simulink model "HW_7_2_1B"  (R2019b)
settings: Solver=VariableStepAuto  StartTime=0.0  StopTime=50  RelTol=1e-3  EnableMultiTasking=on
settings Model: Creator=Teng-Hu  LastModifiedBy=liu
settings DataIOCC: ReturnWorkspaceOutputs=off
settings OptimizationCC: LifeSpan=inf
settings DebuggingCC: SFUnexpectedBacktrackingDiag=warning  SFNoUnconditionalDefaultTransitionDiag=warning  SFExecutionAtInitializationDiag=none  ArithmeticOperatorsInVariantConditions=warning
settings SFSimCC: SimUseLocalCustomCode=off  CustomCodeUndefinedFunction=UseInterfaceOnly
settings RTWCC: RTWUseLocalCustomCode=off
settings CodeAppCC: StateflowObjectComments=on
settings GRTTargetCC: TargetLangStandard=C89/C90 (ANSI)
settings ConfigComp: CovMetricSettings=dw  CovHtmlReporting=on  CovSaveCumulativeToWorkspaceVar=on  CovSaveSingleToWorkspaceVar=on  CovExternalEMLEnable=off

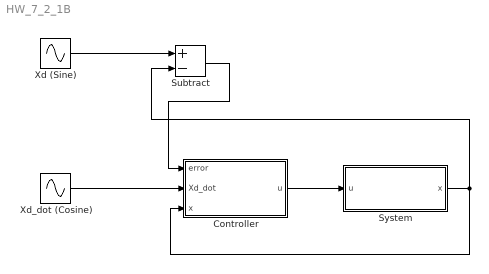
== system HW_7_2_1B ==
  Controller : MATLAB Function  TreatAsAtomicUnit=on
  Subtract : Sum  Inputs=+-
  System : Subsystem
  Xd (Sine) : Sin  SampleTime=0
  Xd_dot (Cosine) : Sin  Phase=pi/2  SampleTime=0
  wires:
  System/1(x) -> Subtract/2, Controller/3(x)
  Subtract/1 -> Controller/1(error)
  Xd (Sine)/1 -> Subtract/1
  Xd_dot (Cosine)/1 -> Controller/2(Xd_dot)
  Controller/1(u) -> System/1(u)

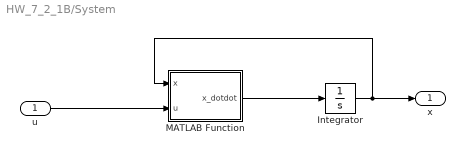
== system HW_7_2_1B/System ==
  u : Inport
  Integrator : Integrator  InitialCondition=1
  MATLAB Function : MATLAB Function  TreatAsAtomicUnit=on
  x : Outport
  wires:
  Integrator/1 -> MATLAB Function/1(x), x/1
  u/1 -> MATLAB Function/2(u)
  MATLAB Function/1(x_dotdot) -> Integrator/1

== matlab function HW_7_2_1B/Controller ==
  data: error input; u output; Xd_dot input; x input
function u = fcn(error, Xd_dot, x)
%#codegen
a = 2;
b = 5;
k = 10;
u = -(a*x+b*cos(x)) + Xd_dot + k*error;

== matlab function HW_7_2_1B/System/MATLAB Function ==
  data: x input; u input; x_dotdot output
function x_dotdot = fcn(x,u)
%#codegen


x_dotdot = 2*x+5*cos(x)+u;
